simulink model "q_3d_crane_test"  (Simulink 6.6)
settings: Solver=FixedStepDiscrete  StartTime=0.0  StopTime=inf  FixedStep=0.001  RelTol=1e-3
values from neighbouring files (symbols this model uses):
  IMAX_AMP = 7    [setup_3d_crane.m]
  K_CURR = -2.0    (= -2)    [config_3d_crane.m]
  K_ENC_ALPHA = 2 * pi / (4 * 1024 )    (= 0.00153398078789)    [config_3d_crane.m]
  K_ENC_GAMMA = 2 * pi / (4 * 1024 )    (= 0.00153398078789)    [config_3d_crane.m]
  K_ENC_THETA = 2 * pi / (4 * 1024 ) / Kg_t    (= 1.53398078789e-05)    [config_3d_crane.m]
  K_ENC_X = - Pt / (4 * 1024 ) / Kg_j    [config_3d_crane.m]
  K_ENC_Z = - 2 * pi * r_y_reel / (4 * 1024 ) / Kg_y    [config_3d_crane.m]
  Ka = 0.5    [config_3d_crane.m]
  VMAX_DAC = 10    [setup_3d_crane.m]
undefined symbols (not defined in the file or in its folder): HIL, qc_get_step_size
libraries: simulink x8, quarc_library x3, simulink_extras x3
settings Model: Creator=MLevis  LastModifiedBy=MLevis  SimulationMode=external  ExtModeTrigDuration=25000
settings SolverCC: PositivePriorityOrder=on
settings RTWCC: SystemTargetFile=quarc_windows.tlc  TemplateMakefile=quarc_default_tmf  Description=QuaRC Win32 Target  ProcessScript=quarc_windows_make_rtw_hook
settings STFCustomTargetCC: TargetFcnLib=ansi_tfl_tmw.mat  TargetPreCompLibLocation=C:\DOCUME~1\ALLUSE~1\APPLIC~1\QUARC\lib\2007a\windows\release  GenFloatMathFcnCalls=ANSI_C  SystemTargetFile=quarc_windows.tlc
settings GRTTargetCC: TargetPreCompLibLocation=C:\DOCUME~1\ALLUSE~1\APPLIC~1\QUARC\lib\2007a\windows\release  MatFileLogging=off  ExtMode=on  ExtModeMexFile=quarc_comm

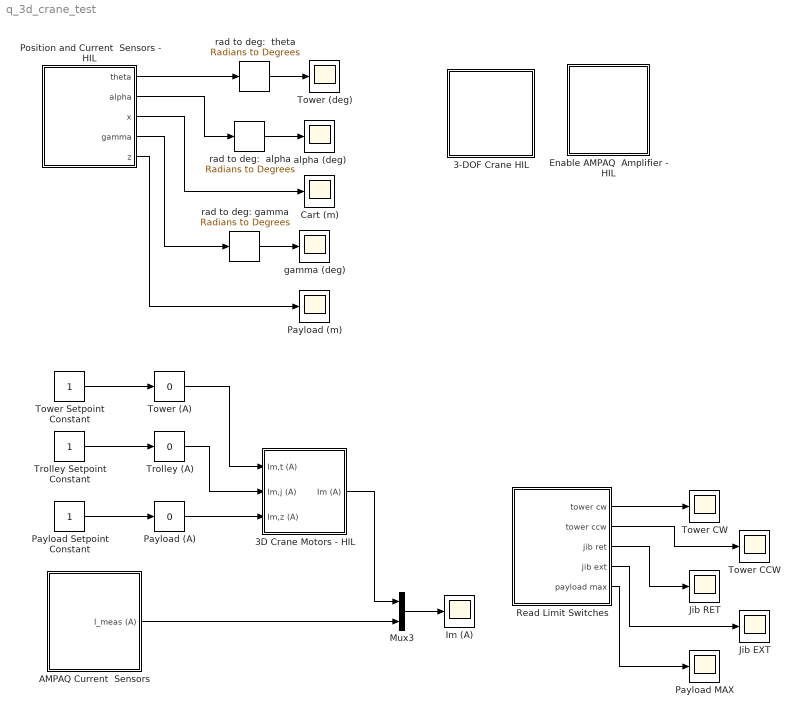
== system q_3d_crane_test ==
  3-DOF Crane HIL : Subsystem
  3D Crane Motors - HIL : Subsystem
  AMPAQ Current  Sensors : Subsystem
  Cart (m) : Scope
      settings: TimeRange=25  YMin=-1  YMax=1  SaveName=ScopeData3
  Enable AMPAQ  Amplifier - HIL : Subsystem
  Im (A) : Scope
  Jib EXT : Scope
      settings: TimeRange=5  YMin=-0.1  YMax=1.1  SaveName=ScopeData9
  Jib RET : Scope
      settings: TimeRange=5  YMin=-0.1  YMax=1.1  SaveName=ScopeData8
  Mux3 : Mux  Inputs=2
  Payload (A) : simulink/Math Operations/Slider Gain  SystemSampleTime=-1  low=-1  gain=0  high=1
  Payload (m) : Scope
      settings: TimeRange=25  YMin=-0.1  YMax=0.9
  Payload MAX : Scope
      settings: TimeRange=5  YMin=-0.1  YMax=1.1  SaveName=ScopeData10
  "Payload Setpoint Constant " : Constant
  Position and Current  Sensors - HIL : Subsystem
  Read Limit Switches : Subsystem
  Tower (A) : simulink/Math Operations/Slider Gain  SystemSampleTime=-1  low=-0.5  gain=0  high=0.5
  Tower (deg) : Scope
      settings: TimeRange=25  YMin=-50  YMax=50  SaveName=ScopeData5
  Tower CCW : Scope
      settings: TimeRange=5  YMin=-0.1  YMax=1.1  SaveName=ScopeData7
  Tower CW : Scope
      settings: TimeRange=5  YMin=-0.1  YMax=1.1  SaveName=ScopeData6
  "Tower Setpoint Constant " : Constant
  Trolley (A) : simulink/Math Operations/Slider Gain  SystemSampleTime=-1  low=-1  gain=0  high=5
  "Trolley Setpoint Constant " : Constant
  alpha (deg) : Scope
      settings: TimeRange=25  YMin=-20  YMax=25  SaveName=ScopeData4
  gamma (deg) : Scope
      settings: TimeRange=25  YMin=-25  YMax=25  SaveName=ScopeData2
  rad to deg:  theta : simulink_extras/Transformations/Radians to Degrees  SystemSampleTime=-1
  rad to deg: gamma : simulink_extras/Transformations/Radians to Degrees  SystemSampleTime=-1
  rad to deg:  alpha : simulink_extras/Transformations/Radians to Degrees  SystemSampleTime=-1
  wires:
  "Tower Setpoint Constant "/1 -> Tower (A)/1
  "Trolley Setpoint Constant "/1 -> Trolley (A)/1
  "Payload Setpoint Constant "/1 -> Payload (A)/1
  Tower (A)/1 -> 3D Crane Motors - HIL/1(Im,t (A))
  Trolley (A)/1 -> 3D Crane Motors - HIL/2(Im,j (A))
  Payload (A)/1 -> 3D Crane Motors - HIL/3(Im,z (A))
  AMPAQ Current  Sensors/1(I_meas (A)) -> Mux3/2
  3D Crane Motors - HIL/1(Im (A)) -> Mux3/1
  Mux3/1 -> Im (A)/1
  rad to deg:  theta/1 -> Tower (deg)/1
  rad to deg:  alpha/1 -> alpha (deg)/1
  rad to deg: gamma/1 -> gamma (deg)/1
  Position and Current  Sensors - HIL/1(theta) -> rad to deg:  theta/1
  Position and Current  Sensors - HIL/2(alpha) -> rad to deg:  alpha/1
  Position and Current  Sensors - HIL/3(x) -> Cart (m)/1
  Position and Current  Sensors - HIL/4(gamma) -> rad to deg: gamma/1
  Position and Current  Sensors - HIL/5(z) -> Payload (m)/1
  Read Limit Switches/1(tower cw) -> Tower CW/1
  Read Limit Switches/2(tower ccw) -> Tower CCW/1
  Read Limit Switches/3(jib ret) -> Jib RET/1
  Read Limit Switches/4(jib ext) -> Jib EXT/1
  Read Limit Switches/5(payload max) -> Payload MAX/1

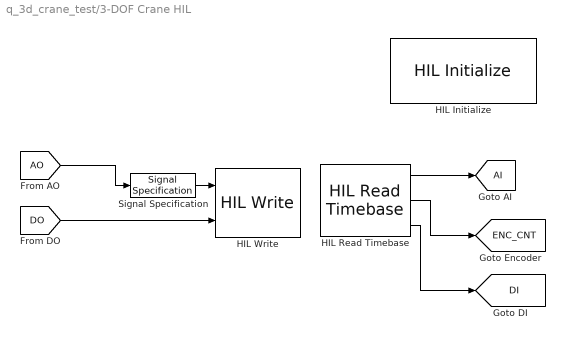
== system q_3d_crane_test/3-DOF Crane HIL ==
  HIL Initialize : quarc_library/Data Acquisition/Generic/Configuration/HIL Initialize  object_name=HIL-1  board_type=q8  board_number=0  exclusive=off  active=on  hardware_clocks=[0:1]  clock_modes=[0 0]  initial_clock_frequencies=[]  set_clock_params_at_start=on  set_clock_params_at_switch_in=off  set_clock_frequencies_at_start=off  set_clock_frequencies_at_switch_in=off  analog_input_channels=[0:7]  analog_input_maximums=10  analog_input_minimums=-10  set_analog_input_params_at_start=off  set_analog_input_params_at_switch_in=off  analog_output_channels=[0:7]  analog_output_maximums=[10]  analog_output_minimums=[-10]  initial_analog_outputs=[0]  final_analog_outputs=[0]  watchdog_analog_outputs=0  set_analog_output_params_at_start=on  set_analog_output_params_at_switch_in=off  set_analog_outputs_at_start=on  set_analog_outputs_at_switch_in=off  set_analog_outputs_at_terminate=on  set_analog_outputs_at_switch_out=off  set_analog_outputs_on_watchdog=off  digital_input_channels=[]  digital_output_channels=[0,1,2,4]  digital_output_configuration=[]  initial_digital_outputs=[1]  final_digital_outputs=[1]  watchdog_digital_outputs=[2]  set_digital_output_params_at_start=off  set_digital_output_params_at_switch_in=off  set_digital_outputs_at_start=on  set_digital_outputs_at_switch_in=off  set_digital_outputs_at_terminate=on  set_digital_outputs_at_switch_out=off  set_digital_outputs_on_watchdog=off  encoder_channels=[0:7]  quadrature=[4]  encoder_filter_frequency=(1/120e-9)/1  initial_encoder_counts=[0]  set_encoder_params_at_start=on  set_encoder_params_at_switch_in=off  set_encoder_counts_at_start=on  set_encoder_counts_at_switch_in=off  pwm_channels=[]  pwm_modes=[0]  pwm_frequency=(1/60e-9)/1024  pwm_configuration=[]  pwm_alignment=[]  pwm_polarity=[]  pwm_leading_deadband=[]  pwm_trailing_deadband=[]  initial_pwm_outputs=[0]  final_pwm_outputs=[0]  watchdog_pwm_outputs=[]  set_pwm_params_at_start=on  set_pwm_params_at_switch_in=off  set_pwm_outputs_at_start=on  set_pwm_outputs_at_switch_in=off  set_pwm_outputs_at_terminate=on  set_pwm_outputs_at_switch_out=off  set_pwm_outputs_on_watchdog=off  other_output_channels=[]  initial_other_outputs=[]  final_other_outputs=[]  watchdog_other_outputs=[]  set_other_outputs_at_start=off  set_other_outputs_at_switch_in=off  set_other_outputs_at_terminate=off  set_other_outputs_at_switch_out=off  set_other_outputs_on_watchdog=off
      settings: AttributesFormatString=%<object_name>
  HIL Read Timebase : quarc_library/Data Acquisition/Generic/Timebases/HIL Read Timebase  Tag=unassigned  object_name=HIL-1  clock=0  analog_channels=[0:2]  encoder_channels=[0:4]  digital_channels=[8:12]  other_channels=[]  samples_in_buffer=max(ceil(1/qc_get_step_size), 1)  active=on  vector_output=on  data_type_mode=Inherit via back propagation  encoder_data_type=double  digital_data_type=boolean
  HIL Write : quarc_library/Data Acquisition/Generic/Immediate I//O/HIL Write  Tag=unassigned  object_name=HIL-1  analog_channels=[0:2]  pwm_channels=[]  digital_channels=[0,1,2,4]  other_channels=[]  sample_time=-1  active=off  vector_input=on
  Signal Specification : SignalSpecification  DataType=double
  tag scope: AI=global, DI=global, ENC_CNT=global
  wires:
  HIL Read Timebase/3 -> [DI]
  HIL Read Timebase/1 -> [AI]
  HIL Read Timebase/2 -> [ENC_CNT]
  [DO] -> HIL Write/2
  [AO] -> Signal Specification/1
  Signal Specification/1 -> HIL Write/1

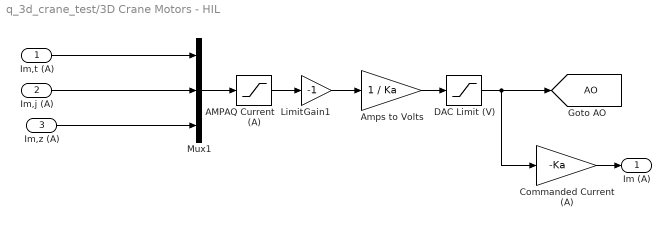
== system q_3d_crane_test/3D Crane Motors - HIL ==
  Im,t (A) : Inport
  Im,j (A) : Inport  Port=2
  Im,z (A) : Inport  Port=3
  AMPAQ Current  Limit (A) : Saturate  UpperLimit=IMAX_AMP  LowerLimit=-IMAX_AMP
  Amps to Volts : Gain  Gain=1 / Ka  SaturateOnIntegerOverflow=on
  Commanded Current (A) : Gain  Gain=-Ka  SaturateOnIntegerOverflow=on
  DAC Limit (V) : Saturate  UpperLimit=VMAX_DAC  LowerLimit=-VMAX_DAC
  Gain1 : Gain  Gain=-1
  Mux1 : Mux  Inputs=3
  Im (A) : Outport
  tag scope: AO=global
  wires:
  Im,z (A)/1 -> Mux1/3
  Im,t (A)/1 -> Mux1/1
  AMPAQ Current  Limit (A)/1 -> Gain1/1
  Mux1/1 -> AMPAQ Current  Limit (A)/1
  DAC Limit (V)/1 -> [AO], Commanded Current (A)/1
  Amps to Volts/1 -> DAC Limit (V)/1
  Im,j (A)/1 -> Mux1/2
  Gain1/1 -> Amps to Volts/1
  Commanded Current (A)/1 -> Im (A)/1

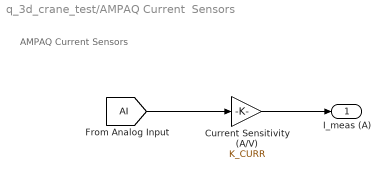
== system q_3d_crane_test/AMPAQ Current  Sensors ==
  note: AMPAQ Current Sensors
  Current Sensitivity (A/V) : Gain  Gain=K_CURR
  I_meas (A) : Outport
  wires:
  Current Sensitivity (A/V)/1 -> I_meas (A)/1
  [AI] -> Current Sensitivity (A/V)/1

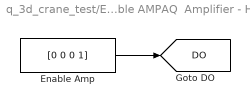
== system q_3d_crane_test/Enable AMPAQ  Amplifier - HIL ==
  Enable Amp : Constant  Value=[0 0 0 1]
  tag scope: DO=global
  wires:
  Enable Amp/1 -> [DO]

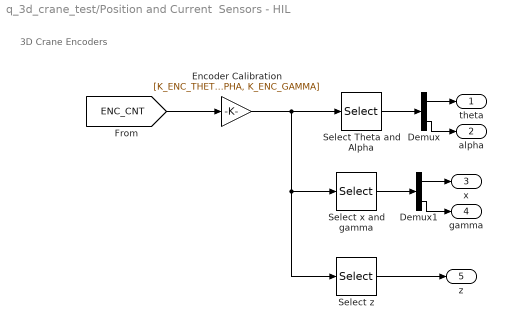
== system q_3d_crane_test/Position and Current  Sensors - HIL ==
  note: 3D Crane Encoders
  Demux : Demux  Outputs=2
  Demux1 : Demux  Outputs=2
  Encoder Calibration : Gain  Gain=[K_ENC_THETA, K_ENC_X, K_ENC_Z, K_ENC_ALPHA, K_ENC_GAMMA]
  Select Theta and Alpha : Selector  IndexOptions=Index vector (dialog)  Indices=[1, 4]  OutputSizes=1  InputPortWidth=5
  Select x and gamma : Selector  IndexOptions=Index vector (dialog)  Indices=[2, 5]  OutputSizes=1  InputPortWidth=5
  Select z : Selector  IndexOptions=Index vector (dialog)  Indices=3  OutputSizes=1  InputPortWidth=5
  theta : Outport
  alpha : Outport  Port=2
  x : Outport  Port=3
  gamma : Outport  Port=4
  z : Outport  Port=5
  wires:
  [ENC_CNT] -> Encoder Calibration/1
  Select Theta and Alpha/1 -> Demux/1
  Select x and gamma/1 -> Demux1/1
  Demux/1 -> theta/1
  Demux/2 -> alpha/1
  Demux1/1 -> x/1
  Demux1/2 -> gamma/1
  Select z/1 -> z/1
  Encoder Calibration/1 -> Select Theta and Alpha/1, Select x and gamma/1, Select z/1

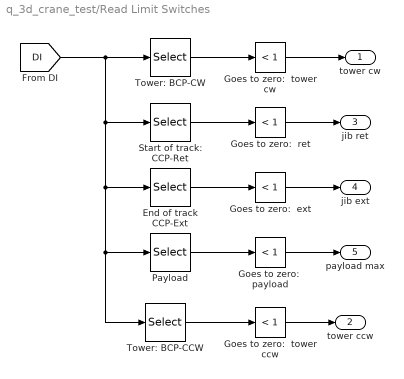
== system q_3d_crane_test/Read Limit Switches ==
  End of track CCP-Ext : Selector  IndexOptions=Index vector (dialog)  Indices=3  OutputSizes=1  InputPortWidth=5
  Goes to zero:  ext : simulink/Logic and Bit Operations/Compare To Constant  SystemSampleTime=-1  relop=<  const=1  LogicOutDataTypeMode=boolean  ZeroCross=off
  Goes to zero:  payload : simulink/Logic and Bit Operations/Compare To Constant  SystemSampleTime=-1  relop=<  const=1  LogicOutDataTypeMode=boolean  ZeroCross=off
  Goes to zero:  ret : simulink/Logic and Bit Operations/Compare To Constant  SystemSampleTime=-1  relop=<  const=1  LogicOutDataTypeMode=boolean  ZeroCross=off
  Goes to zero:  tower ccw : simulink/Logic and Bit Operations/Compare To Constant  SystemSampleTime=-1  relop=<  const=1  LogicOutDataTypeMode=boolean  ZeroCross=off
  Goes to zero:  tower cw : simulink/Logic and Bit Operations/Compare To Constant  SystemSampleTime=-1  relop=<  const=1  LogicOutDataTypeMode=boolean  ZeroCross=off
  Payload : Selector  IndexOptions=Index vector (dialog)  Indices=4  OutputSizes=1  InputPortWidth=5
  Start of track: CCP-Ret : Selector  IndexOptions=Index vector (dialog)  Indices=2  OutputSizes=1  InputPortWidth=5
  Tower: BCP-CCW : Selector  IndexOptions=Index vector (dialog)  Indices=5  OutputSizes=1  InputPortWidth=5
  Tower: BCP-CW : Selector  IndexOptions=Index vector (dialog)  Indices=1  OutputSizes=1  InputPortWidth=5
  tower cw : Outport
  tower ccw : Outport  Port=2
  jib ret : Outport  Port=3
  jib ext : Outport  Port=4
  payload max : Outport  Port=5
  wires:
  [DI] -> End of track CCP-Ext/1, Payload/1, Tower: BCP-CCW/1, Start of track: CCP-Ret/1, Tower: BCP-CW/1
  Payload/1 -> Goes to zero:  payload/1
  Goes to zero:  payload/1 -> payload max/1
  Goes to zero:  tower cw/1 -> tower cw/1
  Tower: BCP-CW/1 -> Goes to zero:  tower cw/1
  Goes to zero:  ret/1 -> jib ret/1
  Goes to zero:  ext/1 -> jib ext/1
  Start of track: CCP-Ret/1 -> Goes to zero:  ret/1
  End of track CCP-Ext/1 -> Goes to zero:  ext/1
  Tower: BCP-CCW/1 -> Goes to zero:  tower ccw/1
  Goes to zero:  tower ccw/1 -> tower ccw/1
